simulink model "RAP4000"  (R2025a)
settings: Solver=VariableStepAuto  StartTime=0.0  StopTime=tspan  RelTol=1e-3
undefined symbols (not defined in the file): CAin, CBin, QA, QB, V
settings DataIOCC: SaveState=on

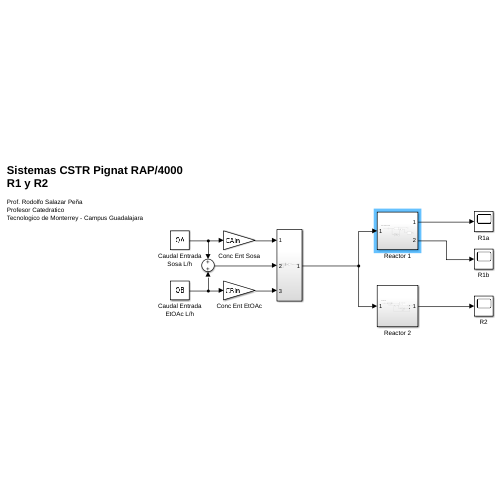
[thumbnail: Simulink's stored preview of the top-level diagram]
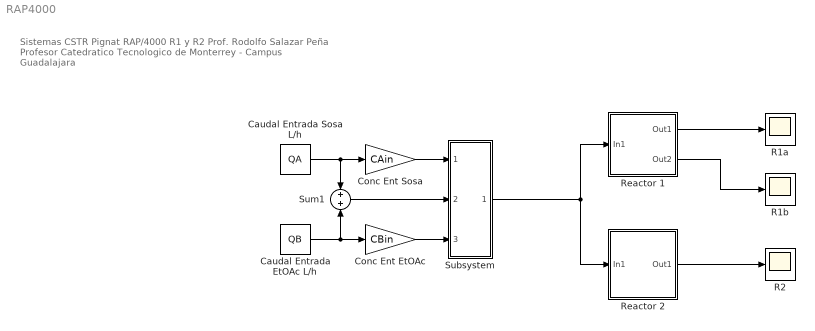
== system RAP4000 ==
  note: Sistemas CSTR Pignat RAP/4000
      | R1 y R2
      |
      | Prof. Rodolfo Salazar Peña
      | Profesor Catedratico
      | Tecnologico de Monterrey - Campus Guadalajara
  Caudal Entrada EtOAc L/h : Constant  Value=QB
  Caudal Entrada Sosa L/h : Constant  Value=QA
  Conc Ent EtOAc : Gain  Gain=CBin
  Conc Ent Sosa : Gain  Gain=CAin
  R1a : Scope
      settings: ActiveDisplayYMinimum=-0.019832384642488463  ActiveDisplayYMaximum=0.17849146178239619
  R1b : Scope
      settings: ActiveDisplayYMinimum=-0.017395328088640777  ActiveDisplayYMaximum=0.15655795279776702
  R2 : Scope
      settings: ActiveDisplayYMinimum=-0.018003419796370285  ActiveDisplayYMaximum=0.16203077816733261  DataLoggingVariableName=ScopeData2
  Reactor 1 : Subsystem
  Reactor 2 : Subsystem
  Subsystem : Subsystem
  Sum1 : Sum
  wires:
  Caudal Entrada Sosa L/h/1 -> Sum1/1, Conc Ent Sosa/1
  Caudal Entrada EtOAc L/h/1 -> Sum1/2, Conc Ent EtOAc/1
  Conc Ent Sosa/1 -> Subsystem/1(In1)
  Sum1/1 -> Subsystem/2(In2)
  Conc Ent EtOAc/1 -> Subsystem/3(In3)
  Subsystem/1(Out1) -> Reactor 2/1(In1), Reactor 1/1(In1)
  Reactor 1/1(Out1) -> R1a/1
  Reactor 1/2(Out2) -> R1b/1
  Reactor 2/1(Out1) -> R2/1

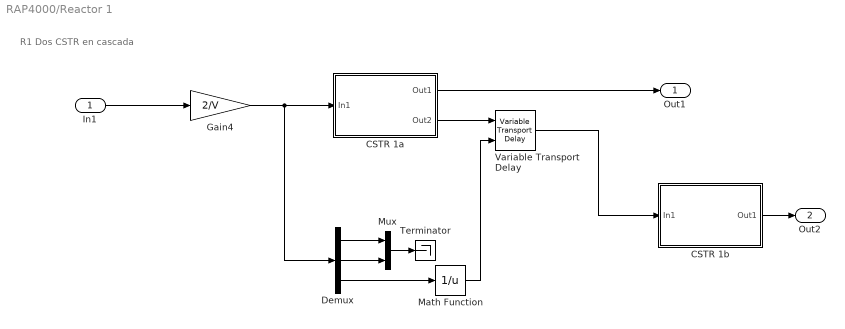
== system RAP4000/Reactor 1 ==
  note: R1 Dos CSTR en cascada
  In1 : Inport
  CSTR 1a : Subsystem
  CSTR 1b : Subsystem
  Demux : Demux  Outputs=3
  Gain4 : Gain  Gain=2/V
  Math Function : Math  Operator=reciprocal
  Mux : Mux  Inputs=2
  Terminator : Terminator
  Variable Transport Delay : VariableTransportDelay  VariableDelayType=Variable transport delay  MaximumDelay=3600
  Out1 : Outport
  Out2 : Outport  Port=2
  wires:
  In1/1 -> Gain4/1
  Gain4/1 -> Demux/1, CSTR 1a/1(In1)
  CSTR 1a/1(Out1) -> Out1/1
  CSTR 1b/1(Out1) -> Out2/1
  CSTR 1a/2(Out2) -> Variable Transport Delay/1
  Variable Transport Delay/1 -> CSTR 1b/1(In1)
  Demux/1 -> Mux/1
  Demux/2 -> Mux/2
  Mux/1 -> Terminator/1
  Demux/3 -> Math Function/1
  Math Function/1 -> Variable Transport Delay/2

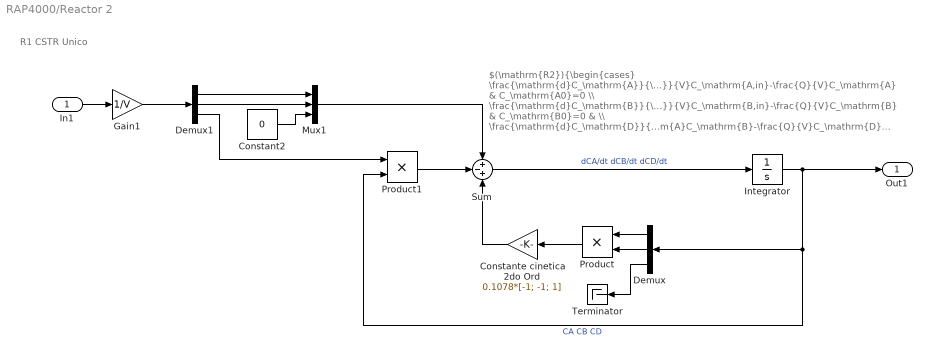
== system RAP4000/Reactor 2 ==
  note: $(\mathrm{R2}){\begin{cases} \frac{\mathrm{d}C_\mathrm{A}}{\mathrm{d}t}=-kC_\mathrm{A}C_\mathrm{B}+\frac{Q_\mathrm{A}}{V}C_\mathrm{A,in}-\frac{Q}{V}C_\mathrm{A} & C_\mathrm{A0}=0 \\ \frac{\mathrm{d}C_\mathrm{B}}{\mathrm{d}t}=-kC_\mathrm{A}C_\mathrm{B}+\frac{Q_\mathrm{B}}{V}C_\mathrm{B,in}-\frac{Q}{V}C_\mathrm{B} & C_\mathrm{B0}=0 & \\ \frac{\mathrm{d}C_\mathrm{D}}{\mathrm{d}t}=kC_\mathrm{A}C_\mathrm{B}-\frac{Q}{V}C_\mathrm{D} & C_\mathrm{D0}=0 & \\ \end{cases}$
  note: R1 CSTR Unico
  In1 : Inport
  Constant2 : Constant  Value=0
  Constante cinetica 2do Ord : Gain  Gain=0.1078*[-1; -1; 1]
  Demux : Demux  Outputs=3
  Demux1 : Demux  Outputs=3
  Gain1 : Gain  Gain=1/V
  Integrator : Integrator  InitialCondition=[0; 0; 0]
  Mux1 : Mux  Inputs=3
  Product : Product
  Product1 : Product
  Sum : Sum  Inputs=+-+
  Terminator : Terminator
  Out1 : Outport
  wires:
  Constante cinetica 2do Ord/1 -> Sum/3
  In1/1 -> Gain1/1
  Demux/1 -> Product/1
  Demux1/3 -> Product1/1
  Demux/3 -> Terminator/1
  Demux1/2 -> Mux1/2
  Demux/2 -> Product/2
  Integrator/1 -> Out1/1, Demux/1, Product1/2  "CA CB CD"
  Mux1/1 -> Sum/1
  Product1/1 -> Sum/2
  Constant2/1 -> Mux1/3
  Product/1 -> Constante cinetica 2do Ord/1
  Demux1/1 -> Mux1/1
  Sum/1 -> Integrator/1  "dCA/dt dCB/dt dCD/dt"
  Gain1/1 -> Demux1/1

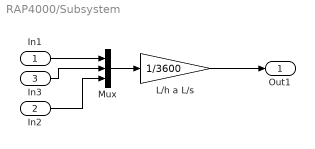
== system RAP4000/Subsystem ==
  In1 : Inport
  In2 : Inport  Port=2
  In3 : Inport  Port=3
  L/h a L/s : Gain  Gain=1/3600
  Mux : Mux  Inputs=3
  Out1 : Outport
  wires:
  Mux/1 -> L/h a L/s/1
  In1/1 -> Mux/1
  L/h a L/s/1 -> Out1/1
  In3/1 -> Mux/2
  In2/1 -> Mux/3

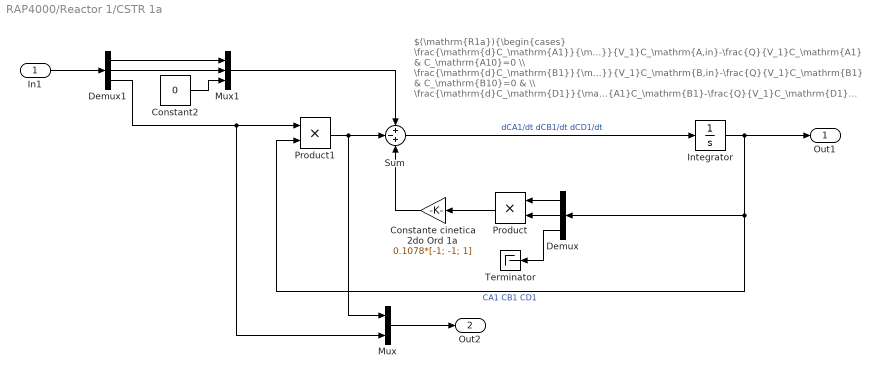
== system RAP4000/Reactor 1/CSTR 1a ==
  note: $(\mathrm{R1a}){\begin{cases} \frac{\mathrm{d}C_\mathrm{A1}}{\mathrm{d}t}=-kC_\mathrm{A1}C_\mathrm{B1}+\frac{Q_\mathrm{A}}{V_1}C_\mathrm{A,in}-\frac{Q}{V_1}C_\mathrm{A1} & C_\mathrm{A10}=0 \\ \frac{\mathrm{d}C_\mathrm{B1}}{\mathrm{d}t}=-kC_\mathrm{A1}C_\mathrm{B1}+\frac{Q_\mathrm{B}}{V_1}C_\mathrm{B,in}-\frac{Q}{V_1}C_\mathrm{B1} & C_\mathrm{B10}=0 & \\ \frac{\mathrm{d}C_\mathrm{D1}}{\mathrm{d}t}=kC_\mathrm{A1}C_\mathrm{B1}-\frac{Q}{V_1}C_\mathrm{D1} & C_\mathrm{D10}=0 & \\ \end{cases}$
  In1 : Inport
  Constant2 : Constant  Value=0
  Constante cinetica 2do Ord 1a : Gain  Gain=0.1078*[-1; -1; 1]
  Demux : Demux  Outputs=3
  Demux1 : Demux  Outputs=3
  Integrator : Integrator  InitialCondition=[0; 0; 0]
  Mux : Mux  Inputs=2
  Mux1 : Mux  Inputs=3
  Product : Product
  Product1 : Product
  Sum : Sum  Inputs=+-+
  Terminator : Terminator
  Out1 : Outport
  Out2 : Outport  Port=2
  wires:
  Constante cinetica 2do Ord 1a/1 -> Sum/3
  In1/1 -> Demux1/1
  Demux/1 -> Product/1
  Demux1/3 -> Mux/2, Product1/1
  Demux/3 -> Terminator/1
  Demux1/2 -> Mux1/2
  Demux/2 -> Product/2
  Integrator/1 -> Out1/1, Demux/1, Product1/2  "CA1 CB1 CD1"
  Mux1/1 -> Sum/1
  Product1/1 -> Mux/1, Sum/2
  Constant2/1 -> Mux1/3
  Product/1 -> Constante cinetica 2do Ord 1a/1
  Demux1/1 -> Mux1/1
  Sum/1 -> Integrator/1  "dCA1/dt dCB1/dt dCD1/dt"
  Mux/1 -> Out2/1

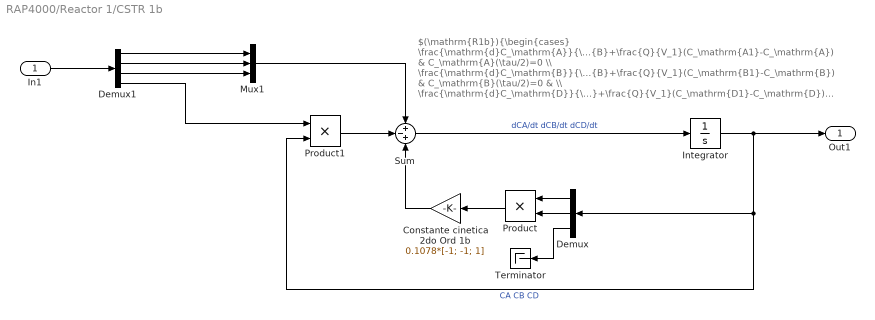
== system RAP4000/Reactor 1/CSTR 1b ==
  note: $(\mathrm{R1b}){\begin{cases} \frac{\mathrm{d}C_\mathrm{A}}{\mathrm{d}t}=-kC_\mathrm{A}C_\mathrm{B}+\frac{Q}{V_1}(C_\mathrm{A1}-C_\mathrm{A}) & C_\mathrm{A}(\tau/2)=0 \\ \frac{\mathrm{d}C_\mathrm{B}}{\mathrm{d}t}=-kC_\mathrm{A}C_\mathrm{B}+\frac{Q}{V_1}(C_\mathrm{B1}-C_\mathrm{B}) & C_\mathrm{B}(\tau/2)=0 & \\ \frac{\mathrm{d}C_\mathrm{D}}{\mathrm{d}t}=kC_\mathrm{A}C_\mathrm{B}+\frac{Q}{V_1}(C_\mathrm{D1}-C_\mathrm{D}) & C_\mathrm{D}(\tau/2)=0 & \\ \end{cases}$
  In1 : Inport
  Constante cinetica 2do Ord 1b : Gain  Gain=0.1078*[-1; -1; 1]
  Demux : Demux  Outputs=3
  Demux1 : Demux
  Integrator : Integrator  InitialCondition=[0; 0; 0]
  Mux1 : Mux  Inputs=3
  Product : Product
  Product1 : Product
  Sum : Sum  Inputs=+-+
  Terminator : Terminator
  Out1 : Outport
  wires:
  Constante cinetica 2do Ord 1b/1 -> Sum/3
  In1/1 -> Demux1/1
  Demux/1 -> Product/1
  Demux/3 -> Terminator/1
  Demux1/2 -> Mux1/2
  Demux/2 -> Product/2
  Integrator/1 -> Out1/1, Demux/1, Product1/2  "CA CB CD"
  Mux1/1 -> Sum/1
  Product1/1 -> Sum/2
  Product/1 -> Constante cinetica 2do Ord 1b/1
  Demux1/1 -> Mux1/1
  Sum/1 -> Integrator/1  "dCA/dt dCB/dt dCD/dt"
  Demux1/3 -> Mux1/3
  Demux1/4 -> Product1/1
